simulink model "motorModel"  (R2021b)
settings: Solver=VariableStepAuto  StartTime=0.0  StopTime=10  RelTol=1e-3
model workspace (MATLAB code in the model file):
  | J=0.018256; b=0.168599; kt=1.595349; kb=1.56749; R=1.746171;L =0;
libraries: fl_lib x5, nesl_utility x5, ee_lib x2, simulink x1
settings Model: Creator=min  LastModifiedBy=min

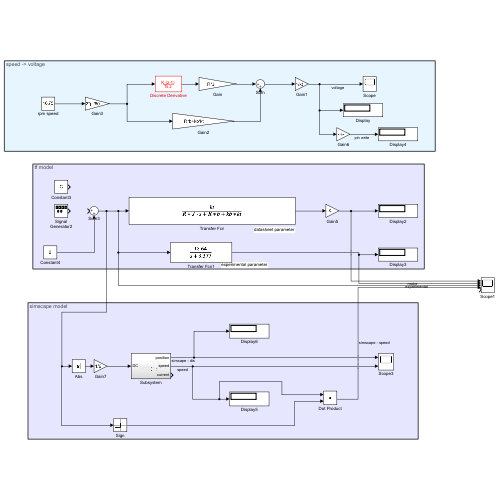
[thumbnail: Simulink's stored preview of the top-level diagram]
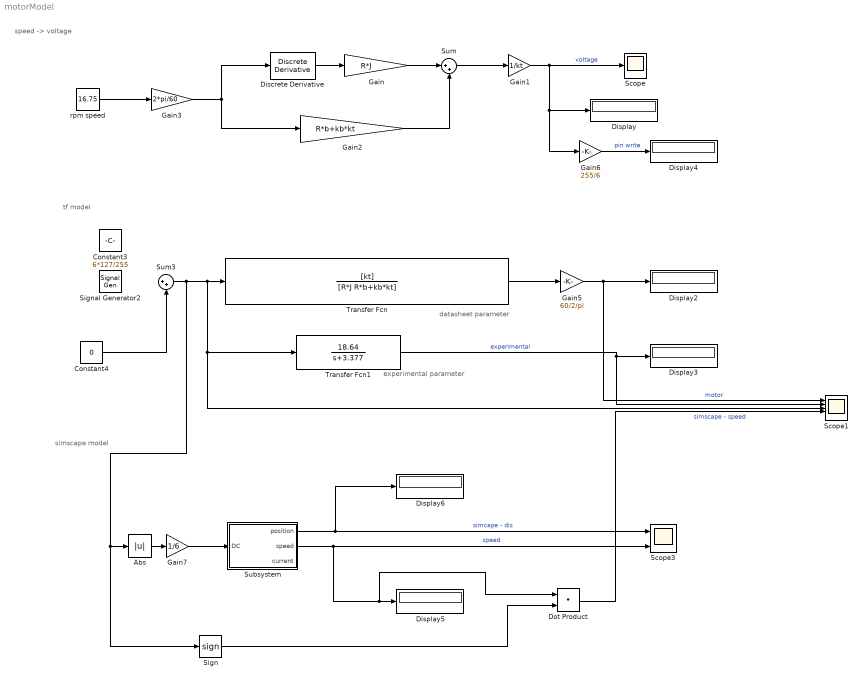
== system motorModel ==
  note: speed -> voltage
  note: datasheet parameter
  note: tf model
  note: simscape model
  note: experimental parameter
  Abs : Abs
  Constant3 : Constant  Value=6*127/255
  Constant4 : Constant  Value=0
  Discrete Derivative : simulink/Discrete/Discrete Derivative  gainval=1.0  ICPrevScaledInput=0.0  OutMin=[]  OutMax=[]  OutDataType=fixdt(1, 16)  OutScaling=2^-10  DoSatur=off
  Display{,2..6} (6 alike) : Display
  Dot Product : DotProduct  InputSameDT=on  OutDataTypeStr=Inherit: Inherit via internal rule
  Gain : Gain  Gain=R*J
  Gain1 : Gain  Gain=1/kt
  Gain2 : Gain  Gain=R*b+kb*kt
  Gain3 : Gain  Gain=2*pi/60
  Gain5 : Gain  Gain=60/2/pi
  Gain6 : Gain  Gain=255/6
  Gain7 : Gain  Gain=1/6
  Scope : Scope
  Scope1 : Scope  NumInputPorts=5
  Scope3 : Scope  NumInputPorts=2
  Sign : Signum
  Signal Generator2 : SignalGenerator  WaveForm=square  Amplitude=6*177/255  Frequency=.3
  Subsystem : Subsystem
  Sum : Sum  Inputs=|++
  Sum3 : Sum  Inputs=|++
  Transfer Fcn : TransferFcn  Numerator=[kt]  Denominator=[R*J R*b+kb*kt]
  Transfer Fcn1 : TransferFcn  Numerator=[18.64]  Denominator=[1 3.377]
  rpm speed : Constant  Value=16.75
  wires:
  Discrete Derivative/1 -> Gain/1
  Sum/1 -> Gain1/1
  Gain/1 -> Sum/1
  Gain2/1 -> Sum/2
  Gain1/1 -> Display/1, Gain6/1, Scope/1  "voltage"
  Gain3/1 -> Gain2/1, Discrete Derivative/1
  rpm speed/1 -> Gain3/1
  Transfer Fcn/1 -> Gain5/1
  Gain5/1 -> Display2/1, Scope1/1  "motor"
  Transfer Fcn1/1 -> Display3/1, Scope1/2  "experimental"
  Sum3/1 -> Sign/1, Abs/1, Transfer Fcn1/1, Scope1/3, Transfer Fcn/1
  Constant4/1 -> Sum3/2
  Gain6/1 -> Display4/1  "pin write"
  Subsystem/1(position) -> Display6/1, Scope3/1  "simcape - dis"
  Subsystem/2(speed) -> Scope3/2, Dot Product/1, Display5/1  "speed"
  Gain7/1 -> Subsystem/1(DC)
  Abs/1 -> Gain7/1
  Sign/1 -> Dot Product/2
  Dot Product/1 -> Scope1/4  "simscape - speed"

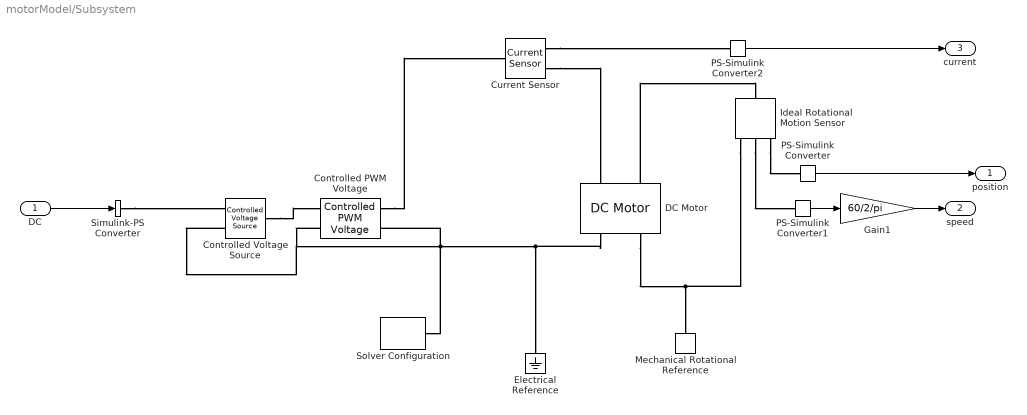
== system motorModel/Subsystem ==
  DC : Inport
  Controlled PWM Voltage : ee_lib/Integrated Circuits/Controlled PWM Voltage  F=1000 Hz  TD=0 s  pulse_width_offset=0 s  pulse_min=0 s  pwm_or_av=1  event_type=1  sample_time=1e-6 s  Vmin=0 V  Vmax=1 V  Vm=6 V  u_min=0  u_max=1
  Controlled Voltage Source : fl_lib/Electrical/Electrical Sources/Controlled Voltage Source
  Current Sensor : fl_lib/Electrical/Electrical Sensors/Current Sensor
  DC Motor : ee_lib/Electromechanical/Brushed Motors/DC Motor  field_option=ee.enum.field_option.pm  Rf=100 Ohm  Lf=1 H  Laf=0.15 H  If0=0 A  parameterization=ee.enum.dcparam_option.circuit_param  Ra=R Ohm  La=L H  emf_or_torque=ee.enum.emf_or_torque.kv  Kv=kb V/(rad/s)  Ki=6.876e-4 N*m/A  T_stall=0.24e-3 N*m  w_max=19100 rpm  w_rated=15000 rpm  P_rated=0.08 W  V_rated=1.5 V  lam_param=ee.enum.lam_param.damping  i_noload=0 A  V_i_noload=1.5 V  J=J kg*m^2  lam=b N*m/(rad/s)  speed0=0 rpm  enable_fault_armature=simscape.enum.onoff.off  rev_faulted=1 / 3  G_faulted_armature=1e-5 S  fault_trigger_armature=ee.enum.faults.faultTrigger.temporal  t_fault_armature=1 s  max_permissible_current_armature=inf A  t_fail_on_current_armature=1 s  enable_fault_field=simscape.enum.onoff.off  G_faulted_field=1e-5 S  fault_trigger_field=ee.enum.faults.faultTrigger.temporal  t_fault_field=1 s  max_permissible_current_field=inf A  t_fail_on_current_field=1 s  fault_action=simscape.enum.assert.action.none  alpha=3.93e-3 1/K  Tmeas=25 degC  thermal_mass=100 J/K  initial_temperature=25 degC
  Electrical Reference : fl_lib/Electrical/Electrical Elements/Electrical Reference
  Gain1 : Gain  Gain=60/2/pi
  Ideal Rotational Motion Sensor : fl_lib/Mechanical/Mechanical Sensors/Ideal Rotational Motion Sensor  wrap_angle=simscape.enum.onoff.off  offset=0 rad
  Mechanical Rotational Reference : fl_lib/Mechanical/Rotational Elements/Mechanical Rotational Reference
  PS-Simulink Converter : nesl_utility/PS-Simulink Converter  PhysicalDomain=network_engine_domain  SubClassName=ps_output  LeftPortType=input  RightPortType=output  PseudoPeriodic=off  Frequencies=[]  Unit=inherit  AffineConversion=off
      settings: SourceProductBaseCode=PW,SS
  PS-Simulink Converter1 : nesl_utility/PS-Simulink Converter  PhysicalDomain=network_engine_domain  SubClassName=ps_output  LeftPortType=input  RightPortType=output  PseudoPeriodic=off  Frequencies=[]  Unit=inherit  AffineConversion=off
      settings: SourceProductBaseCode=PW,SS
  PS-Simulink Converter2 : nesl_utility/PS-Simulink Converter  PhysicalDomain=network_engine_domain  SubClassName=ps_output  LeftPortType=input  RightPortType=output  PseudoPeriodic=off  Frequencies=[]  Unit=inherit  AffineConversion=off
      settings: SourceProductBaseCode=PW,SS
  Simulink-PS Converter : nesl_utility/Simulink-PS Converter  PhysicalDomain=network_engine_domain  SubClassName=ps_input  LeftPortType=input  RightPortType=output  PseudoPeriodic=off  Frequencies=[]  NoiseDistribution=none  NoiseParameters=[]  Unit=1  AffineConversion=off  FilteringAndDerivatives=provide  SimscapeFilterOrder=1  InputFilterTimeConstant=0.001  UdotUserProvided=0
      settings: SourceProductBaseCode=PW,SS
  Solver Configuration : nesl_utility/Solver Configuration  PhysicalDomain=network_engine_domain  SubClassName=solver  LeftPortType=input  RightPortType=generic  Tones=[]  Harmonics=[]  SimulateNoise=off  Profile=off  UseLocalSampling=off  EnableSwitchedLinearOptims=on  FrequencyDomain=off  UseCCode=off  RelTol=0.001  AbsTol=1e-06  MinStep=1e-09  ToWorkspace=off  RevertToSquareIcSolve=off  NumHomotopyIterations=100  PhasorMode=off  PhasorModeNumHarmonics=1  DoDC=off  ResidualTolerance=1e-09  UseLocalSolver=off  LocalSolverChoice=NE_BACKWARD_EULER_ADVANCER  LocalSolverSampleTime=0.001  DoFixedCost=off  MaxNonlinIter=3  MaxModeIter=2  ComputeImpulses=off  ImpulseIterations=2  LinearAlgebra=auto  EquationFormulation=NE_TIME_EF  DelaysMemoryBudget=1024  AutomaticFiltering=on  FilteringTimeConstant=0.001  PartitionStorageMethod=AS_NEEDED  PartitionMemoryBudget=1024  PartitionMethod=ROBUST
      settings: SourceProductBaseCode=PW,SS
  position : Outport
  speed : Outport  Port=2
  current : Outport  Port=3
  wires:
  PS-Simulink Converter1/1 -> Gain1/1
  Gain1/1 -> speed/1
  PS-Simulink Converter2/1 -> current/1
  PS-Simulink Converter/1 -> position/1
  DC/1 -> Simulink-PS Converter/1
  connections:
  DC Motor/LConn2 -- Ideal Rotational Motion Sensor/LConn1
  DC Motor/RConn2 -- Ideal Rotational Motion Sensor/RConn1 -- Mechanical Rotational Reference/LConn1
  Solver Configuration/RConn1 -- Controlled Voltage Source/RConn2 -- Controlled PWM Voltage/LConn2 -- Controlled PWM Voltage/RConn2 -- DC Motor/RConn1 -- Electrical Reference/LConn1
  Controlled PWM Voltage/RConn1 -- Current Sensor/LConn1
  Current Sensor/RConn2 -- DC Motor/LConn1
  Ideal Rotational Motion Sensor/RConn3 -- PS-Simulink Converter/LConn1
  Ideal Rotational Motion Sensor/RConn2 -- PS-Simulink Converter1/LConn1
  Current Sensor/RConn1 -- PS-Simulink Converter2/LConn1
  Simulink-PS Converter/RConn1 -- Controlled Voltage Source/RConn1
  Controlled Voltage Source/LConn1 -- Controlled PWM Voltage/LConn1
